simulink model "Sliding_Mode_Observer_Sensorless"  (R2020a)
settings: Solver=ode45  StartTime=0.0  StopTime=0.7  MaxStep=5e-6  RelTol=1e-3
values from neighbouring files (symbols this model uses):
  f = -R/Ld    (= -633.333333333)    [NC_controllers.m]
  fpwm = 20e3    (= 20000)    [NC_controllers.m]
  g = 1/Ld    (= 333.333333333)    [NC_controllers.m]
  inertia = 1.8e-4    (= 0.00018)    [NC_controllers.m]
  ki = (-5.135 + 5.347)/Ts    (= 4240)    [NC_controllers.m]
  Ki_est = w_n^2    (= 98696.0440109)    [NC_controllers.m]
  Ki_speed = (alphas/2/zeta)^2*inertia    [NC_controllers.m]
  kp = 5.347    [NC_controllers.m]
  Kp_est = 2*zeta*w_n    (= 628.318530718)    [NC_controllers.m]
  Kp_speed = alphas*inertia    [NC_controllers.m]
  Ld = 3e-3    (= 0.003)    [NC_controllers.m]
  Lq = 3e-3    (= 0.003)    [NC_controllers.m]
  LT = 2.8    [NC_controllers.m]
  p = 4    [NC_controllers.m]
  phi_PM = 0.1    [NC_controllers.m]
  R = 1.9    [NC_controllers.m]
  ramp_rate = 5    [NC_controllers.m]
  speedFilter_freq = 75    [NC_controllers.m]
  Ts = 1/fpwm    (= 5e-05)    [NC_controllers.m]
  Tspeed = Ts*10/10    (= 5e-05)    [NC_controllers.m]
  Vdc = 450    [NC_controllers.m]
  wm = 2*pi*ff    (= 1675.51608191)    [NC_controllers.m]
libraries: simulink x5
settings Model: Creator=Nicky  LastModifiedBy=Nicky
settings DebuggingCC: ArithmeticOperatorsInVariantConditions=warning
settings SFSimCC: CustomCodeUndefinedFunction=UseInterfaceOnly
settings CodeAppCC: StateflowObjectComments=on

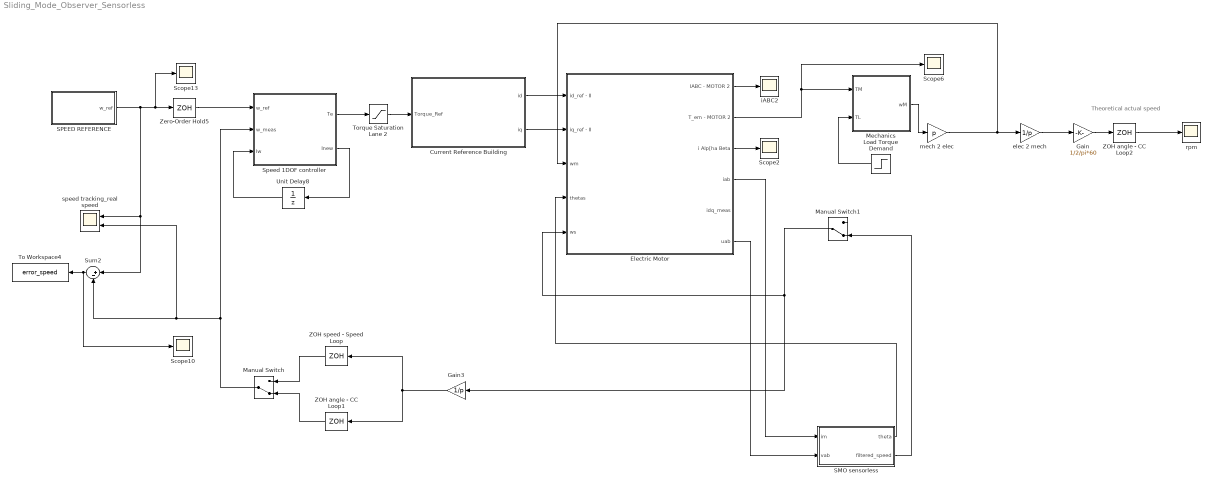
== system Sliding_Mode_Observer_Sensorless ==
  note: Theoretical actual speed
  Current Reference Building : Subsystem
  Electric Motor : Subsystem
  Gain : Gain  Gain=1/2/pi*60
  Gain3 : Gain  Gain=1/p
  Load Torque Demand : Step  Time=0.4  After=LT  SampleTime=0
  Manual Switch : ManualSwitch  CurrentSetting=0
  Manual Switch1 : ManualSwitch  CurrentSetting=0
  Mechanics : Subsystem
  SMO sensorless : Subsystem
  "SPEED REFERENCE " : Subsystem
  Scope{2,6,10,13} (4 alike) : Scope
  Speed 1DOF controller : MATLAB Function  TreatAsAtomicUnit=on
  Sum2 : Sum  Inputs=|+-
  To Workspace4 : ToWorkspace  VariableName=error_speed  SaveFormat=Timeseries  SampleTime=-1
      settings: Decimation=10
  Torque Saturation Lane 2 : Saturate  UpperLimit=10  LowerLimit=-10
  Unit Delay8 : UnitDelay  SampleTime=Ts  HasFrameUpgradeWarning=on
  ZOH angle - CC Loop1 : ZeroOrderHold  SampleTime=Ts
  ZOH angle - CC Loop2 : ZeroOrderHold  SampleTime=Ts
  ZOH speed - Speed Loop : ZeroOrderHold  SampleTime=Tspeed
  Zero-Order Hold5 : ZeroOrderHold  SampleTime=Tspeed
  elec 2 mech : Gain  Gain=1/p
  iABC2 : Scope
  mech 2 elec : Gain  Gain=p
  rpm : Scope
  speed tracking_real speed : Scope  NumInputPorts=2
  wires:
  Mechanics/1(wM) -> mech 2 elec/1
  Load Torque Demand/1 -> Mechanics/2(TL)
  "SPEED REFERENCE "/1(w_ref) -> Scope13/1, Zero-Order Hold5/1, Sum2/1, speed tracking_real speed/1
  Sum2/1 -> Scope10/1, To Workspace4/1
  Electric Motor/1(IABC - MOTOR 2) -> iABC2/1
  Manual Switch/1 -> Speed 1DOF controller/2(w_meas), speed tracking_real speed/2, Sum2/2
  Speed 1DOF controller/1(Te) -> Torque Saturation Lane 2/1
  Zero-Order Hold5/1 -> Speed 1DOF controller/1(w_ref)
  Torque Saturation Lane 2/1 -> Current Reference Building/1(Torque_Ref)
  Electric Motor/3(i Alp[ha Beta) -> Scope2/1
  Gain/1 -> ZOH angle - CC Loop2/1
  elec 2 mech/1 -> Gain/1
  ZOH angle - CC Loop2/1 -> rpm/1
  Unit Delay8/1 -> Speed 1DOF controller/3(Iw)
  Speed 1DOF controller/2(Inew) -> Unit Delay8/1
  ZOH angle - CC Loop1/1 -> Manual Switch/2
  ZOH speed - Speed Loop/1 -> Manual Switch/1
  Electric Motor/2(T_em - MOTOR 2) -> Mechanics/1(TM), Scope6/1
  Current Reference Building/1(id) -> Electric Motor/1(id_ref - II)
  Current Reference Building/2(iq) -> Electric Motor/2(iq_ref - II)
  Gain3/1 -> ZOH speed - Speed Loop/1, ZOH angle - CC Loop1/1
  mech 2 elec/1 -> Electric Motor/3(wm), elec 2 mech/1
  Manual Switch1/1 -> Gain3/1, Electric Motor/5(ws)
  Electric Motor/4(iab) -> SMO sensorless/1(im)
  Electric Motor/6("uab ") -> SMO sensorless/2(vab)
  SMO sensorless/1(theta) -> Electric Motor/4(thetas)
  SMO sensorless/2(filtered_speed) -> Manual Switch1/2

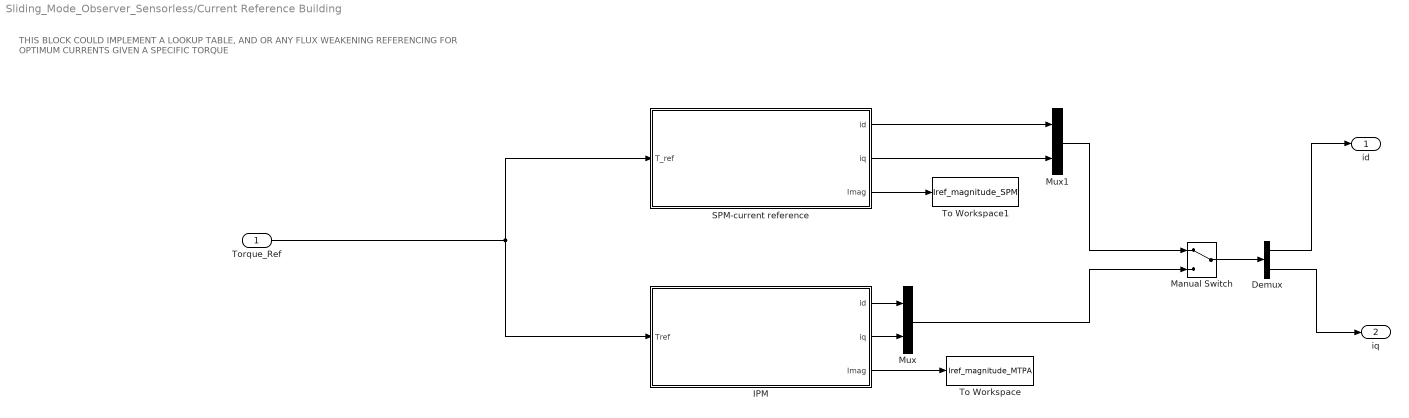
== system Sliding_Mode_Observer_Sensorless/Current Reference Building ==
  note: THIS BLOCK COULD IMPLEMENT A LOOKUP TABLE, AND OR ANY FLUX WEAKENING REFERENCING FOR OPTIMUM CURRENTS GIVEN A SPECIFIC TORQUE
  Torque_Ref : Inport
  Demux : Demux  Outputs=2
  IPM : MATLAB Function  TreatAsAtomicUnit=on
  Manual Switch : ManualSwitch
  Mux : Mux  Inputs=2
  Mux1 : Mux  Inputs=2
  SPM-current reference : MATLAB Function  TreatAsAtomicUnit=on
  To Workspace : ToWorkspace  VariableName=Iref_magnitude_MTPA  SaveFormat=Timeseries  SampleTime=-1
      settings: Decimation=10
  To Workspace1 : ToWorkspace  VariableName=Iref_magnitude_SPM  SaveFormat=Timeseries  SampleTime=-1
      settings: Decimation=10
  id : Outport  VectorParamsAs1DForOutWhenUnconnected=off
  iq : Outport  Port=2  VectorParamsAs1DForOutWhenUnconnected=off
  wires:
  SPM-current reference/1(id) -> Mux1/1
  SPM-current reference/2(iq) -> Mux1/2
  Demux/1 -> id/1
  Demux/2 -> iq/1
  Manual Switch/1 -> Demux/1
  IPM/2(iq) -> Mux/2
  IPM/1(id) -> Mux/1
  Mux1/1 -> Manual Switch/1
  Mux/1 -> Manual Switch/2
  IPM/3(Imag) -> To Workspace/1
  SPM-current reference/3(Imag) -> To Workspace1/1
  Torque_Ref/1 -> IPM/1(Tref), SPM-current reference/1(T_ref)

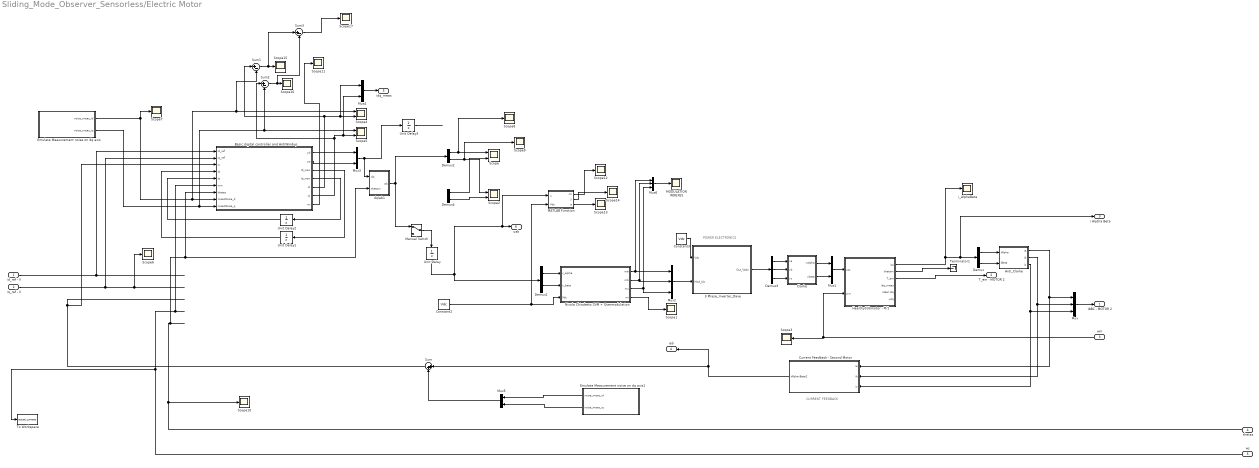
== system Sliding_Mode_Observer_Sensorless/Electric Motor ==
  note: CURRENT FEEDBACK
  note: POWER ELECTRONICS
  id_ref - II : Inport
  iq_ref - II : Inport  Port=2
  wm : Inport  Port=3
  thetas : Inport  Port=4
  ws : Inport  Port=5
  3 Phase_Inverter_Dave : Subsystem
  Anti_Clarke : Subsystem
  Basic digital controller and AntiWindup : MATLAB Function  TreatAsAtomicUnit=on
  Clarke : Subsystem
  Constant2 : Constant  Value=Vdc
  Constant3 : Constant  Value=Vdc
  Current Feedback - Second Motor : Subsystem
  Demux{,1..2,4} (4 alike) : Demux  Outputs=2
  Demux3 : Demux  Outputs=3
  Emulate Measurement noise on dq axis : Subsystem
  Emulate Measurement noise on dq axis1 : Subsystem
  HealthySUbmotor - PI/1 : Subsystem
  MATLAB Function : MATLAB Function  TreatAsAtomicUnit=on
  MODULATION INDEXES : Scope
  Manual Switch : ManualSwitch
  Mux : Mux  Inputs=3
  Mux{1,3..5} (4 alike) : Mux  Inputs=2
  Mux2 : Mux  Inputs=3
  Mux6 : Mux  Inputs=3
  Nicola Chiodetto SVM + Overmodulation : MATLAB Function  TreatAsAtomicUnit=on
  Scope{,2,4..5} (4 alike) : Scope  NumInputPorts=2
  Scope{1,3,6..17} (14 alike) : Scope
  Sum : Sum  Inputs=|++
  Sum1 : Sum  Inputs=|+-
  Sum2 : Sum  Inputs=|+-
  Sum3 : Sum  Inputs=|+-
  Terminator1 : Terminator
  To Workspace : ToWorkspace  VariableName=actual_currents  SaveFormat=Timeseries  SampleTime=-1
  Unit Delay{,1..3} (4 alike) : UnitDelay  SampleTime=1/fpwm  HasFrameUpgradeWarning=on
  dq/ab1 : Subsystem
  i_AlphaBeta : Scope
  IABC - MOTOR 2 : Outport  VectorParamsAs1DForOutWhenUnconnected=off
  T_em - MOTOR 2 : Outport  Port=2  VectorParamsAs1DForOutWhenUnconnected=off
  i Alp[ha Beta : Outport  Port=3  VectorParamsAs1DForOutWhenUnconnected=off
  iab : Outport  Port=4  VectorParamsAs1DForOutWhenUnconnected=off
  idq_meas : Outport  Port=5  VectorParamsAs1DForOutWhenUnconnected=off
  "uab " : Outport  Port=6  VectorParamsAs1DForOutWhenUnconnected=off
  wires:
  HealthySUbmotor - PI/1/1(iss) -> Demux/1, i Alp[ha Beta/1, i_AlphaBeta/1
  Anti_Clarke/3(ic) -> Current Feedback - Second Motor/3(ic), Mux/3
  Demux3/1 -> Clarke/1(va)
  Clarke/2(vbeta) -> Mux1/2
  iq_ref - II/1 -> Basic digital controller and AntiWindup/2(iq_ref), Scope6/1
  Clarke/1(valpha) -> Mux1/1
  Demux/2 -> Anti_Clarke/2(iBeta)
  ? -> Demux4/1, Manual Switch/2
  Anti_Clarke/2(ib) -> Current Feedback - Second Motor/2(ib), Mux/2
  Constant3/1 -> 3 Phase_Inverter_Dave/1(Vdc)
  ws/1 -> Basic digital controller and AntiWindup/6(wm), To Workspace/1
  Demux/1 -> Anti_Clarke/1(iAlpha)
  Demux3/2 -> Clarke/2(vb)
  Mux2/1 -> 3 Phase_Inverter_Dave/2(Mod_Idx)
  HealthySUbmotor - PI/1/2(thetam) -> Terminator1/1
  Mux6/1 -> MODULATION INDEXES/1
  Demux1/1 -> Nicola Chiodetto SVM + Overmodulation/1(v_alpha)
  Demux1/2 -> Nicola Chiodetto SVM + Overmodulation/2(v_beta)
  Demux3/3 -> Clarke/3(vc)
  Nicola Chiodetto SVM + Overmodulation/4(mi) -> Scope1/1
  HealthySUbmotor - PI/1/3(T_em) -> T_em - MOTOR 2/1
  wm/1 -> HealthySUbmotor - PI/1/2(wm), Scope3/1
  Nicola Chiodetto SVM + Overmodulation/1(ma) -> Mux2/1, Mux6/1
  Mux/1 -> IABC - MOTOR 2/1
  Nicola Chiodetto SVM + Overmodulation/2(mb) -> Mux2/2, Mux6/2
  Nicola Chiodetto SVM + Overmodulation/3(mc) -> Mux2/3, Mux6/3
  Current Feedback - Second Motor/1(iAlpha-Beta2) -> iab/1, Sum/1
  Anti_Clarke/1(ia) -> Current Feedback - Second Motor/1(ia), Mux/1
  Mux1/1 -> HealthySUbmotor - PI/1/1(uss)
  3 Phase_Inverter_Dave/1(Out_Vabc) -> Demux3/1
  Basic digital controller and AntiWindup/1(yd) -> Mux3/1
  Basic digital controller and AntiWindup/2(yq) -> Mux3/2
  Mux3/1 -> Unit Delay3/1, dq/ab1/1(dq)
  Basic digital controller and AntiWindup/3(Id_new) -> Unit Delay1/1
  Unit Delay1/1 -> Basic digital controller and AntiWindup/4(Id)
  Basic digital controller and AntiWindup/4(Iq_new) -> Unit Delay2/1
  Unit Delay2/1 -> Basic digital controller and AntiWindup/5(Iq)
  id_ref - II/1 -> Basic digital controller and AntiWindup/1(id_ref)
  dq/ab1/1(ab) -> Demux2/1, Manual Switch/1
  Manual Switch/1 -> Unit Delay/1
  Demux2/1 -> Scope8/1, Scope/1
  Demux4/1 -> Scope/2
  Demux2/2 -> Scope9/1, Scope2/1
  Demux4/2 -> Scope2/2
  thetas/1 -> Scope10/1, dq/ab1/2(thetam), Basic digital controller and AntiWindup/7(thetas)
  Basic digital controller and AntiWindup/5(id) -> Sum1/1, Mux4/1, Scope4/2
  Basic digital controller and AntiWindup/6(iq) -> Sum2/1, Mux4/2, Scope5/2
  ? -> ?
  Emulate Measurement noise on dq axis/1(noise_meas_id) -> Scope7/1, Sum1/2, Scope4/1, Basic digital controller and AntiWindup/8(measNoise_d)
  Mux4/1 -> idq_meas/1
  Emulate Measurement noise on dq axis/2(noise_meas_iq) -> Sum2/2, Scope5/1, Basic digital controller and AntiWindup/9(measNoise_q)
  Unit Delay3/1 -> ?
  Emulate Measurement noise on dq axis1/1(noise_meas_id) -> Mux5/1
  Emulate Measurement noise on dq axis1/2(noise_meas_iq) -> Mux5/2
  Sum/1 -> Basic digital controller and AntiWindup/3(is)
  Mux5/1 -> Sum/2
  Unit Delay/1 -> Demux1/1, MATLAB Function/1(u), "uab "/1
  Constant2/1 -> MATLAB Function/2(Vdc), Nicola Chiodetto SVM + Overmodulation/3(Vdc)
  Basic digital controller and AntiWindup/7(mi) -> Scope11/1
  MATLAB Function/1(mi) -> Scope12/1
  MATLAB Function/3(a) -> Scope13/1
  MATLAB Function/2(y) -> Scope14/1
  Sum1/1 -> Sum3/1, Scope15/1
  Sum2/1 -> Sum3/2, Scope16/1
  Sum3/1 -> Scope17/1

== system Sliding_Mode_Observer_Sensorless/Mechanics ==
  TM : Inport
  TL : Inport  Port=2
  Gain : Gain  Gain=1/inertia  SaturateOnIntegerOverflow=on  OutDataTypeStr=Inherit: Same as input  ParamDataTypeStr=Inherit: Same as input
  Integrator : Integrator
  Sum : Sum  Inputs=|+-  InputSameDT=on  SaturateOnIntegerOverflow=on  OutDataTypeStr=Inherit: Same as first input
  wM : Outport  VectorParamsAs1DForOutWhenUnconnected=off
  wires:
  TL/1 -> Sum/2
  Sum/1 -> Gain/1
  Gain/1 -> Integrator/1
  Integrator/1 -> wM/1
  TM/1 -> Sum/1

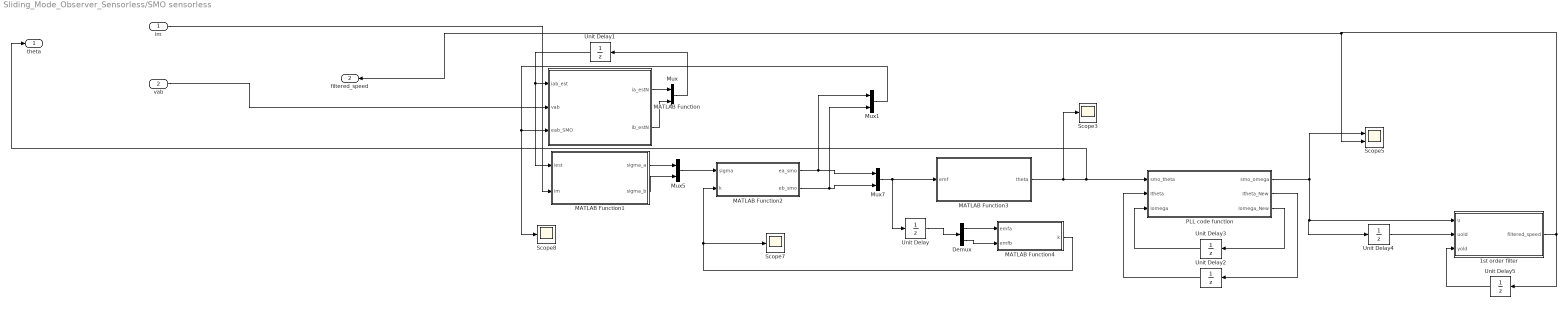
== system Sliding_Mode_Observer_Sensorless/SMO sensorless ==
  im : Inport
  vab : Inport  Port=2
  1st order filter : MATLAB Function  TreatAsAtomicUnit=on
  Demux : Demux  Outputs=2
  MATLAB Function : MATLAB Function  TreatAsAtomicUnit=on
  MATLAB Function1 : MATLAB Function  TreatAsAtomicUnit=on
  MATLAB Function2 : MATLAB Function  TreatAsAtomicUnit=on
  MATLAB Function3 : MATLAB Function  TreatAsAtomicUnit=on
  MATLAB Function4 : MATLAB Function  TreatAsAtomicUnit=on
  Mux{,1,5,7} (4 alike) : Mux  Inputs=2
  PLL code function : MATLAB Function  TreatAsAtomicUnit=on
  Scope3 : Scope
  Scope5 : Scope  NumInputPorts=2
  Scope7 : Scope
  Scope8 : Scope
  Unit Delay{,2..5} (5 alike) : UnitDelay  SampleTime=Ts  HasFrameUpgradeWarning=on
  Unit Delay1 : UnitDelay  InitialCondition=[0; 0]  SampleTime=Ts  HasFrameUpgradeWarning=on
  theta : Outport
  filtered_speed : Outport  Port=2
  wires:
  Unit Delay2/1 -> PLL code function/2(Itheta)
  Unit Delay/1 -> Demux/1
  MATLAB Function1/2(sigma_b) -> Mux5/2
  Unit Delay4/1 -> 1st order filter/2(uold)
  PLL code function/1(smo_omega) -> Scope5/1, Unit Delay4/1, 1st order filter/1(u)
  Mux7/1 -> Unit Delay/1, MATLAB Function3/1(emf)
  Mux1/1 -> MATLAB Function/3(eab_SMO), Scope8/1
  PLL code function/2(Itheta_New) -> Unit Delay2/1
  MATLAB Function/1(ia_estN) -> Mux/1
  Demux/2 -> MATLAB Function4/2(emfb)
  MATLAB Function2/2(eb_smo) -> Mux1/2, Mux7/2
  MATLAB Function/2(ib_estN) -> Mux/2
  Mux5/1 -> MATLAB Function2/1(sigma)
  MATLAB Function2/1(ea_smo) -> Mux1/1, Mux7/1
  Demux/1 -> MATLAB Function4/1(emfa)
  1st order filter/1(filtered_speed) -> filtered_speed/1, Scope5/2, Unit Delay5/1
  PLL code function/3(Iomega_New) -> Unit Delay3/1
  Unit Delay1/1 -> MATLAB Function1/1(iest), MATLAB Function/1(iab_est)
  Mux/1 -> Unit Delay1/1
  MATLAB Function1/1(sigma_a) -> Mux5/1
  MATLAB Function3/1(theta) -> Scope3/1, theta/1, PLL code function/1(smo_theta)
  Unit Delay5/1 -> 1st order filter/3(yold)
  im/1 -> MATLAB Function1/2(im)
  MATLAB Function4/1(k) -> Scope7/1, MATLAB Function2/2(k)
  vab/1 -> MATLAB Function/2(vab)
  Unit Delay3/1 -> PLL code function/3(Iomega)

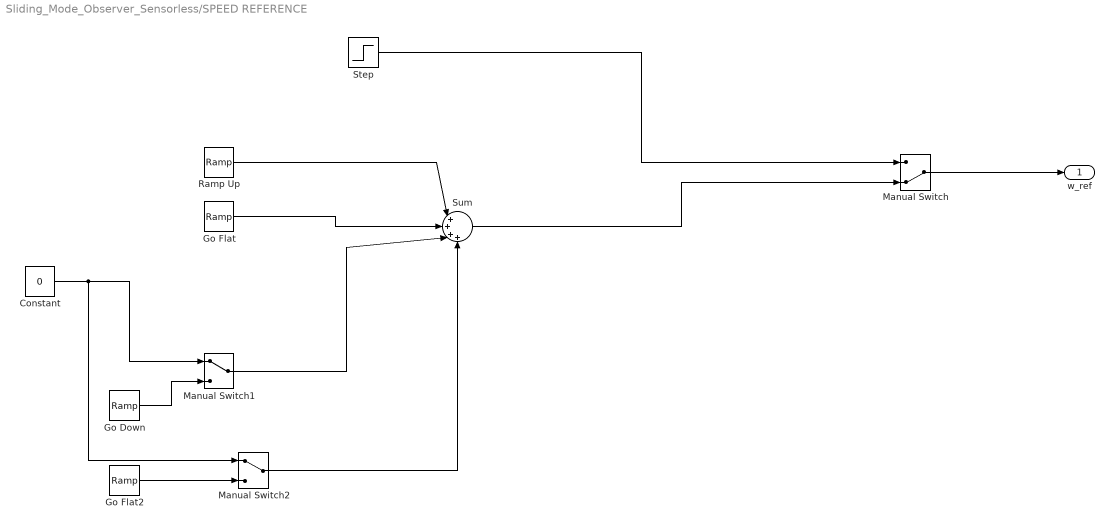
== system Sliding_Mode_Observer_Sensorless/SPEED REFERENCE  ==
  Constant : Constant  Value=0
  Go Down : simulink/Sources/Ramp  slope=-ramp_rate*wm/p  start=0.5  InitialOutput=0
  Go Flat : simulink/Sources/Ramp  slope=-ramp_rate*wm/p  start=1/ramp_rate  InitialOutput=0
  Go Flat2 : simulink/Sources/Ramp  slope=ramp_rate*wm/p  start=0.5+1/ramp_rate  InitialOutput=0
  Manual Switch : ManualSwitch  CurrentSetting=0
  Manual Switch1 : ManualSwitch
  Manual Switch2 : ManualSwitch
  Ramp Up : simulink/Sources/Ramp  slope=ramp_rate*wm/p  start=0  InitialOutput=0
  Step : Step  Time=0.05  After=wm/p  SampleTime=0
  Sum : Sum  Inputs=|++++
  w_ref : Outport  VectorParamsAs1DForOutWhenUnconnected=off
  wires:
  Ramp Up/1 -> Sum/1
  Step/1 -> Manual Switch/1
  Manual Switch/1 -> w_ref/1
  Sum/1 -> Manual Switch/2
  Go Flat/1 -> Sum/2
  Manual Switch1/1 -> Sum/3
  Go Down/1 -> Manual Switch1/2
  Constant/1 -> Manual Switch2/1, Manual Switch1/1
  Go Flat2/1 -> Manual Switch2/2
  Manual Switch2/1 -> Sum/4

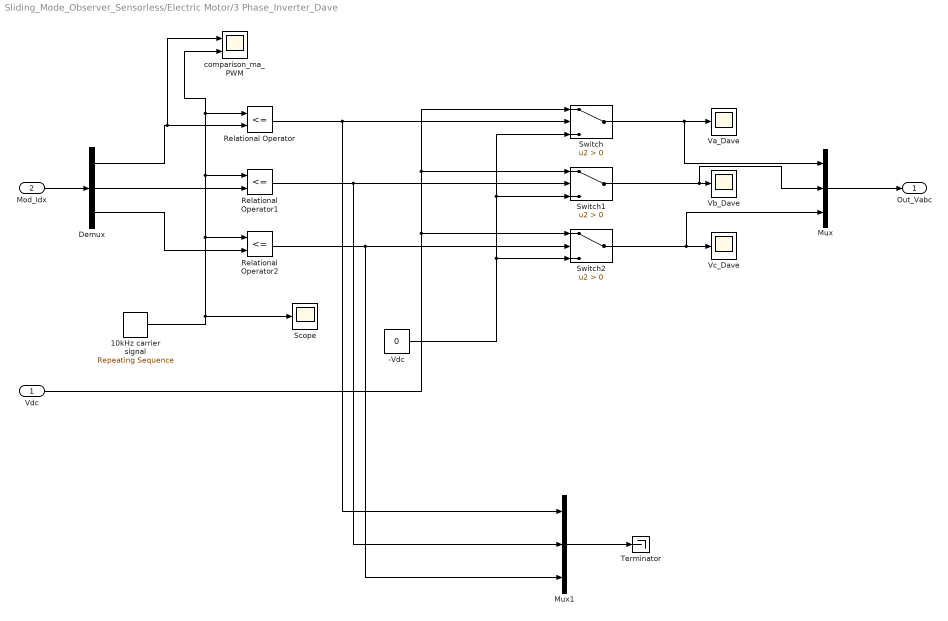
== system Sliding_Mode_Observer_Sensorless/Electric Motor/3 Phase_Inverter_Dave ==
  Vdc : Inport
  Mod_Idx : Inport  Port=2
  -Vdc : Constant  Value=0
  10kHz carrier signal : simulink/Sources/Repeating Sequence  rep_seq_t=[0 .5*Ts Ts]  rep_seq_y="[1  0 1]"
  Demux : Demux  Outputs=3
  Mux : Mux  Inputs=3
  Mux1 : Mux  Inputs=3
  Relational Operator : RelationalOperator  Operator=<=  OutDataTypeStr=boolean  RndMeth=Nearest
  Relational Operator1 : RelationalOperator  Operator=<=  OutDataTypeStr=boolean  RndMeth=Nearest
  Relational Operator2 : RelationalOperator  Operator=<=  OutDataTypeStr=boolean  RndMeth=Nearest
  Scope : Scope
  Switch : Switch  Criteria=u2 > Threshold
  Switch1 : Switch  Criteria=u2 > Threshold
  Switch2 : Switch  Criteria=u2 > Threshold
  Terminator : Terminator
  Va_Dave : Scope
  Vb_Dave : Scope
  Vc_Dave : Scope
  comparison_ma_PWM : Scope  NumInputPorts=2
  Out_Vabc : Outport  VectorParamsAs1DForOutWhenUnconnected=off
  wires:
  Vdc/1 -> Switch2/1, Switch1/1, Switch/1
  -Vdc/1 -> Switch2/3, Switch1/3, Switch/3
  Switch/1 -> Mux/1, Va_Dave/1
  Switch2/1 -> Mux/3, Vc_Dave/1
  Relational Operator2/1 -> Mux1/3, Switch2/2
  Relational Operator1/1 -> Mux1/2, Switch1/2
  10kHz carrier signal/1 -> Scope/1, Relational Operator1/1, comparison_ma_PWM/2, Relational Operator/1, Relational Operator2/1
  Demux/1 -> comparison_ma_PWM/1, Relational Operator/2
  Mod_Idx/1 -> Demux/1
  Demux/3 -> Relational Operator2/2
  Demux/2 -> Relational Operator1/2
  Relational Operator/1 -> Mux1/1, Switch/2
  Mux/1 -> Out_Vabc/1
  Switch1/1 -> Mux/2, Vb_Dave/1
  Mux1/1 -> Terminator/1

== system Sliding_Mode_Observer_Sensorless/Electric Motor/Anti_Clarke ==
  iAlpha : Inport
  iBeta : Inport  Port=2
  " root3/2" : Gain  Gain=0.86602540378443864676372317075294  SaturateOnIntegerOverflow=on  OutDataTypeStr=Inherit: Same as input  ParamDataTypeStr=Inherit: Same as input
  1/2 : Gain  Gain=1/2  SaturateOnIntegerOverflow=on  OutDataTypeStr=Inherit: Same as input  ParamDataTypeStr=Inherit: Same as input
  Sum2 : Sum  Inputs=--  InputSameDT=on  SaturateOnIntegerOverflow=on  OutDataTypeStr=Inherit: Same as first input
  Sum4 : Sum  Inputs=-+  InputSameDT=on  SaturateOnIntegerOverflow=on  OutDataTypeStr=Inherit: Same as first input
  ia : Outport  VectorParamsAs1DForOutWhenUnconnected=off
  ib : Outport  Port=2  VectorParamsAs1DForOutWhenUnconnected=off
  ic : Outport  Port=3  VectorParamsAs1DForOutWhenUnconnected=off
  wires:
  iBeta/1 -> " root3/2"/1
  " root3/2"/1 -> Sum4/2, Sum2/2
  1/2/1 -> Sum2/1, Sum4/1
  Sum2/1 -> ic/1
  Sum4/1 -> ib/1
  iAlpha/1 -> 1/2/1, ia/1

== system Sliding_Mode_Observer_Sensorless/Electric Motor/Clarke ==
  va : Inport
  vb : Inport  Port=2
  vc : Inport  Port=3
  " " : Gain  Gain=2/3  SaturateOnIntegerOverflow=on  OutDataTypeStr=Inherit: Same as input  ParamDataTypeStr=Inherit: Same as input
  "   " : Gain  Gain=1/3  SaturateOnIntegerOverflow=on  OutDataTypeStr=Inherit: Same as input  ParamDataTypeStr=Inherit: Same as input
  "    " : Gain  Gain=1/3  SaturateOnIntegerOverflow=on  OutDataTypeStr=Inherit: Same as input  ParamDataTypeStr=Inherit: Same as input
  " 1/root3" : Gain  Gain=0.57735026918962576450914878050196  SaturateOnIntegerOverflow=on  OutDataTypeStr=Inherit: Same as input  ParamDataTypeStr=Inherit: Same as input
  Sum1 : Sum  Inputs=+-  InputSameDT=on  SaturateOnIntegerOverflow=on  OutDataTypeStr=Inherit: Same as first input
  Sum4 : Sum  Inputs=+--  InputSameDT=on  SaturateOnIntegerOverflow=on  OutDataTypeStr=Inherit: Same as first input
  valpha : Outport  VectorParamsAs1DForOutWhenUnconnected=off
  vbeta : Outport  Port=2  VectorParamsAs1DForOutWhenUnconnected=off
  wires:
  Sum4/1 -> valpha/1
  " "/1 -> Sum4/1
  va/1 -> " "/1
  "    "/1 -> Sum4/2
  "   "/1 -> Sum4/3
  vb/1 -> "    "/1, Sum1/1
  vc/1 -> "   "/1, Sum1/2
  Sum1/1 -> " 1/root3"/1
  " 1/root3"/1 -> vbeta/1

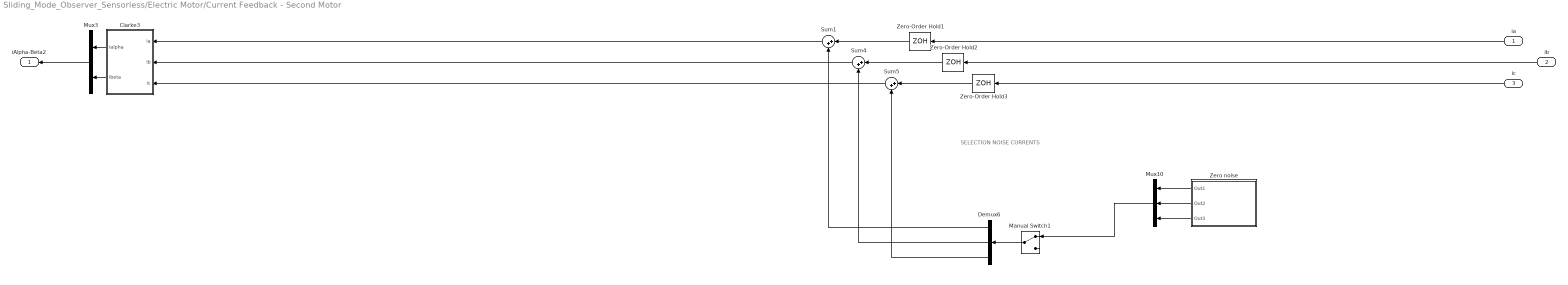
== system Sliding_Mode_Observer_Sensorless/Electric Motor/Current Feedback - Second Motor ==
  note: SELECTION NOISE CURRENTS
  ia : Inport
  ib : Inport  Port=2
  ic : Inport  Port=3
  Clarke3 : Subsystem
  Demux6 : Demux  Outputs=3
  Manual Switch1 : ManualSwitch
  Mux10 : Mux  Inputs=3
  Mux3 : Mux  Inputs=2
  Sum1 : Sum  Inputs=|++
  Sum4 : Sum  Inputs=|++
  Sum5 : Sum  Inputs=|++
  Zero noise : Subsystem
  Zero-Order Hold1 : ZeroOrderHold  SampleTime=1/fpwm
  Zero-Order Hold2 : ZeroOrderHold  SampleTime=1/fpwm
  Zero-Order Hold3 : ZeroOrderHold  SampleTime=1/fpwm
  iAlpha-Beta2 : Outport  VectorParamsAs1DForOutWhenUnconnected=off
  wires:
  Clarke3/1(ialpha) -> Mux3/1
  Demux6/3 -> Sum5/2
  Zero-Order Hold3/1 -> Sum5/1
  Sum4/1 -> Clarke3/2(ib)
  Zero-Order Hold1/1 -> Sum1/1
  Zero-Order Hold2/1 -> Sum4/1
  Mux3/1 -> iAlpha-Beta2/1
  Zero noise/1(Out1) -> Mux10/1
  ia/1 -> Zero-Order Hold1/1
  Sum5/1 -> Clarke3/3(ic)
  Zero noise/2(Out2) -> Mux10/2
  Zero noise/3(Out3) -> Mux10/3
  Demux6/1 -> Sum1/2
  Manual Switch1/1 -> Demux6/1
  Mux10/1 -> Manual Switch1/1
  Demux6/2 -> Sum4/2
  Clarke3/2(ibeta) -> Mux3/2
  ib/1 -> Zero-Order Hold2/1
  ic/1 -> Zero-Order Hold3/1
  Sum1/1 -> Clarke3/1(ia)

== system Sliding_Mode_Observer_Sensorless/Electric Motor/Emulate Measurement noise on dq axis ==
  Constant5 : Constant  Value=0
  Manual Switch : ManualSwitch  CurrentSetting=0
  Manual Switch1 : ManualSwitch
  Zero-Order Hold : ZeroOrderHold  SampleTime=Ts
  Zero-Order Hold1 : ZeroOrderHold  SampleTime=Ts
  noise_meas_id : Outport  VectorParamsAs1DForOutWhenUnconnected=off
  noise_meas_iq : Outport  Port=2  VectorParamsAs1DForOutWhenUnconnected=off
  wires:
  Constant5/1 -> Zero-Order Hold1/1, Zero-Order Hold/1, Manual Switch1/2, Manual Switch/1
  Zero-Order Hold/1 -> Manual Switch/2
  Manual Switch/1 -> noise_meas_id/1
  Zero-Order Hold1/1 -> Manual Switch1/1
  Manual Switch1/1 -> noise_meas_iq/1

== system Sliding_Mode_Observer_Sensorless/Electric Motor/Emulate Measurement noise on dq axis1 ==
  Constant5 : Constant  Value=0
  Manual Switch : ManualSwitch  CurrentSetting=0
  Manual Switch1 : ManualSwitch
  Zero-Order Hold : ZeroOrderHold  SampleTime=Ts
  Zero-Order Hold1 : ZeroOrderHold  SampleTime=Ts
  noise_meas_id : Outport  VectorParamsAs1DForOutWhenUnconnected=off
  noise_meas_iq : Outport  Port=2  VectorParamsAs1DForOutWhenUnconnected=off
  wires:
  Constant5/1 -> Zero-Order Hold1/1, Zero-Order Hold/1, Manual Switch1/2, Manual Switch/1
  Zero-Order Hold/1 -> Manual Switch/2
  Manual Switch/1 -> noise_meas_id/1
  Zero-Order Hold1/1 -> Manual Switch1/1
  Manual Switch1/1 -> noise_meas_iq/1

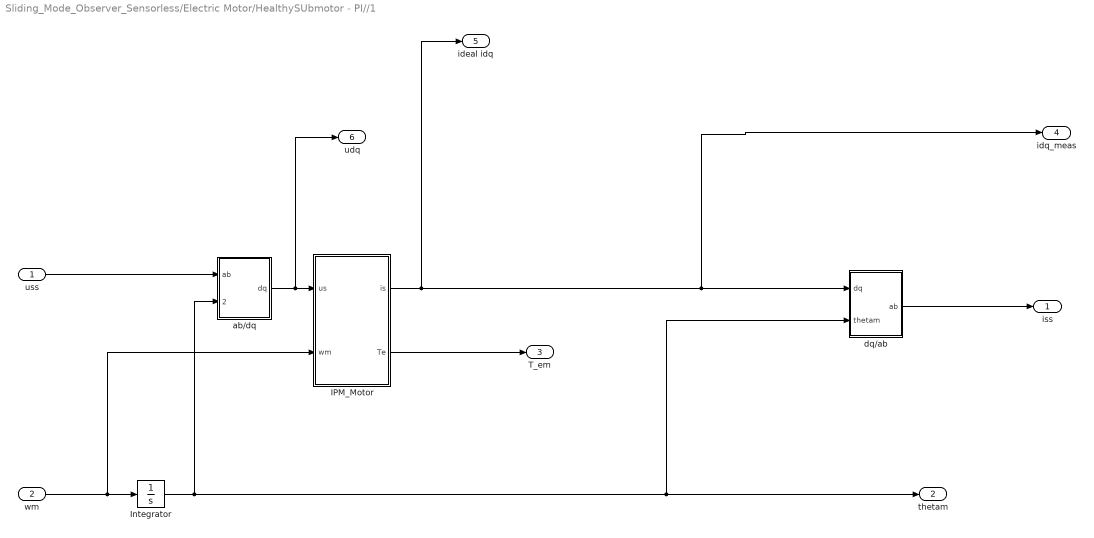
== system Sliding_Mode_Observer_Sensorless/Electric Motor/HealthySUbmotor - PI//1 ==
  uss : Inport
  wm : Inport  Port=2
  IPM_Motor : Subsystem
  Integrator : Integrator
  ab/dq : Subsystem
  dq/ab : Subsystem
  iss : Outport  VectorParamsAs1DForOutWhenUnconnected=off
  thetam : Outport  Port=2  VectorParamsAs1DForOutWhenUnconnected=off
  T_em : Outport  Port=3  VectorParamsAs1DForOutWhenUnconnected=off
  idq_meas : Outport  Port=4  VectorParamsAs1DForOutWhenUnconnected=off
  ideal idq : Outport  Port=5  VectorParamsAs1DForOutWhenUnconnected=off
  udq : Outport  Port=6  VectorParamsAs1DForOutWhenUnconnected=off
  wires:
  uss/1 -> ab/dq/1(ab)
  dq/ab/1(ab) -> iss/1
  IPM_Motor/2(Te) -> T_em/1
  ab/dq/1(dq) -> udq/1, IPM_Motor/1(us)
  wm/1 -> IPM_Motor/2(wm), Integrator/1
  Integrator/1 -> dq/ab/2(thetam), thetam/1, ab/dq/2(thetame)
  IPM_Motor/1(is) -> idq_meas/1, dq/ab/1(dq), ideal idq/1

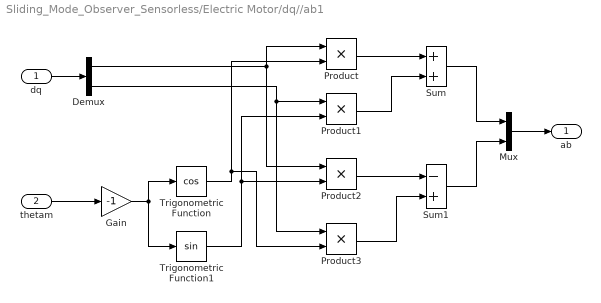
== system Sliding_Mode_Observer_Sensorless/Electric Motor/dq//ab1 ==
  dq : Inport
  thetam : Inport  Port=2
  Demux : Demux  Outputs=2
  Gain : Gain  Gain=-1
  Mux : Mux  Inputs=2
  Product{,1..3} (4 alike) : Product  RndMeth=Zero
  Sum : Sum  InputSameDT=on  SaturateOnIntegerOverflow=on  OutDataTypeStr=Inherit: Same as first input
  Sum1 : Sum  Inputs=-+  InputSameDT=on  SaturateOnIntegerOverflow=on  OutDataTypeStr=Inherit: Same as first input
  Trigonometric Function : Trigonometry  Operator=cos
  Trigonometric Function1 : Trigonometry
  ab : Outport  VectorParamsAs1DForOutWhenUnconnected=off
  wires:
  Product3/1 -> Sum1/2
  Product2/1 -> Sum1/1
  Product1/1 -> Sum/2
  Trigonometric Function1/1 -> Product2/2, Product1/2
  Demux/2 -> Product3/1, Product1/1
  Product/1 -> Sum/1
  Trigonometric Function/1 -> Product3/2, Product/2
  Demux/1 -> Product/1, Product2/1
  Sum1/1 -> Mux/2
  Sum/1 -> Mux/1
  Gain/1 -> Trigonometric Function1/1, Trigonometric Function/1
  thetam/1 -> Gain/1
  dq/1 -> Demux/1
  Mux/1 -> ab/1

== system Sliding_Mode_Observer_Sensorless/Electric Motor/Current Feedback - Second Motor/Clarke3 ==
  ia : Inport
  ib : Inport  Port=2
  ic : Inport  Port=3
  " " : Gain  Gain=2/3  SaturateOnIntegerOverflow=on  OutDataTypeStr=Inherit: Same as input  ParamDataTypeStr=Inherit: Same as input
  "   " : Gain  Gain=1/3  SaturateOnIntegerOverflow=on  OutDataTypeStr=Inherit: Same as input  ParamDataTypeStr=Inherit: Same as input
  "    " : Gain  Gain=1/3  SaturateOnIntegerOverflow=on  OutDataTypeStr=Inherit: Same as input  ParamDataTypeStr=Inherit: Same as input
  " 1/root3" : Gain  Gain=0.57735026918962576450914878050196  SaturateOnIntegerOverflow=on  OutDataTypeStr=Inherit: Same as input  ParamDataTypeStr=Inherit: Same as input
  Sum1 : Sum  Inputs=+-  InputSameDT=on  SaturateOnIntegerOverflow=on  OutDataTypeStr=Inherit: Same as first input
  Sum4 : Sum  Inputs=+--  InputSameDT=on  SaturateOnIntegerOverflow=on  OutDataTypeStr=Inherit: Same as first input
  ialpha : Outport  VectorParamsAs1DForOutWhenUnconnected=off
  ibeta : Outport  Port=2  VectorParamsAs1DForOutWhenUnconnected=off
  wires:
  Sum4/1 -> ialpha/1
  " "/1 -> Sum4/1
  ia/1 -> " "/1
  "    "/1 -> Sum4/2
  "   "/1 -> Sum4/3
  ib/1 -> "    "/1, Sum1/1
  ic/1 -> "   "/1, Sum1/2
  Sum1/1 -> " 1/root3"/1
  " 1/root3"/1 -> ibeta/1

== system Sliding_Mode_Observer_Sensorless/Electric Motor/Current Feedback - Second Motor/Zero noise ==
  Constant : Constant  Value=0
  Constant4 : Constant  Value=0
  Constant5 : Constant  Value=0
  Out1 : Outport  VectorParamsAs1DForOutWhenUnconnected=off
  Out2 : Outport  Port=2  VectorParamsAs1DForOutWhenUnconnected=off
  Out3 : Outport  Port=3  VectorParamsAs1DForOutWhenUnconnected=off
  wires:
  Constant/1 -> Out2/1
  Constant4/1 -> Out3/1
  Constant5/1 -> Out1/1

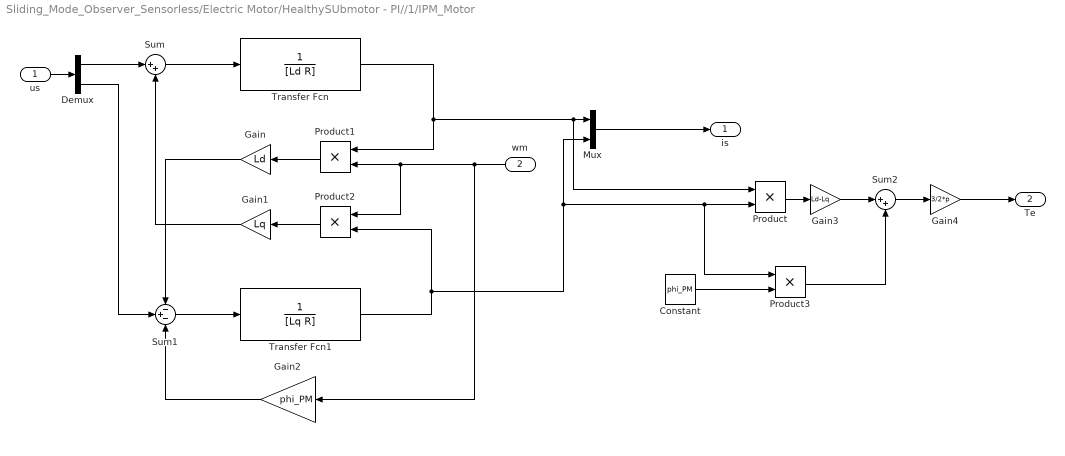
== system Sliding_Mode_Observer_Sensorless/Electric Motor/HealthySUbmotor - PI//1/IPM_Motor ==
  us : Inport
  wm : Inport  Port=2
  Constant : Constant  Value=phi_PM
  Demux : Demux  Outputs=2
  Gain : Gain  Gain=Ld
  Gain1 : Gain  Gain=Lq
  Gain2 : Gain  Gain=phi_PM
  Gain3 : Gain  Gain=Ld-Lq
  Gain4 : Gain  Gain=3/2*p
  Mux : Mux  Inputs=2
  Product{,1..3} (4 alike) : Product
  Sum : Sum  Inputs=|++
  Sum1 : Sum  Inputs=-+-
  Sum2 : Sum  Inputs=|++
  Transfer Fcn : TransferFcn  Denominator=[Ld R]
  Transfer Fcn1 : TransferFcn  Denominator=[Lq R]
  is : Outport  VectorParamsAs1DForOutWhenUnconnected=off
  Te : Outport  Port=2  VectorParamsAs1DForOutWhenUnconnected=off
  wires:
  us/1 -> Demux/1
  Demux/1 -> Sum/1
  Sum/1 -> Transfer Fcn/1
  Transfer Fcn/1 -> Product/1, Mux/1, Product1/1
  wm/1 -> Gain2/1, Product2/1, Product1/2
  Product1/1 -> Gain/1
  Product2/1 -> Gain1/1
  Gain1/1 -> Sum/2
  Gain/1 -> Sum1/1
  Sum1/1 -> Transfer Fcn1/1
  Demux/2 -> Sum1/2
  Transfer Fcn1/1 -> Product2/2, Product3/1, Product/2, Mux/2
  Gain2/1 -> Sum1/3
  Mux/1 -> is/1
  Product/1 -> Gain3/1
  Gain3/1 -> Sum2/1
  Sum2/1 -> Gain4/1
  Product3/1 -> Sum2/2
  Gain4/1 -> Te/1
  Constant/1 -> Product3/2

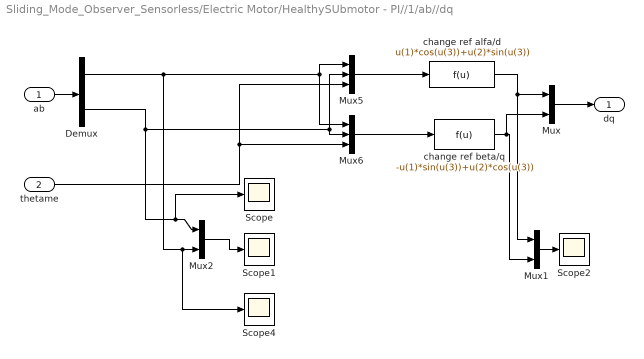
== system Sliding_Mode_Observer_Sensorless/Electric Motor/HealthySUbmotor - PI//1/ab//dq ==
  ab : Inport
  thetame : Inport  Port=2
  Demux : Demux  Outputs=2
  Mux : Mux  Inputs=2
  Mux1 : Mux  Inputs=2
  Mux2 : Mux  Inputs=2
  Mux5 : Mux  Inputs=3
  Mux6 : Mux  Inputs=3
  Scope{,1..2,4} (4 alike) : Scope
  change ref alfa/d : Fcn  Expr=u(1)*cos(u(3))+u(2)*sin(u(3))
  change ref beta/q : Fcn  Expr=-u(1)*sin(u(3))+u(2)*cos(u(3))
  dq : Outport  VectorParamsAs1DForOutWhenUnconnected=off
  wires:
  Demux/1 -> Scope4/1, Mux2/2, Mux5/1, Mux6/1
  Demux/2 -> Scope/1, Mux2/1, Mux6/2, Mux5/2
  thetame/1 -> Mux6/3, Mux5/3
  change ref alfa/d/1 -> Mux/1, Mux1/1
  change ref beta/q/1 -> Mux/2, Mux1/2
  Mux2/1 -> Scope1/1
  Mux1/1 -> Scope2/1
  ab/1 -> Demux/1
  Mux/1 -> dq/1
  Mux5/1 -> change ref alfa/d/1
  Mux6/1 -> change ref beta/q/1

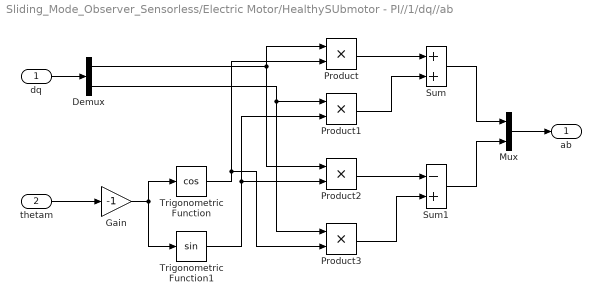
== system Sliding_Mode_Observer_Sensorless/Electric Motor/HealthySUbmotor - PI//1/dq//ab ==
  dq : Inport
  thetam : Inport  Port=2
  Demux : Demux  Outputs=2
  Gain : Gain  Gain=-1
  Mux : Mux  Inputs=2
  Product{,1..3} (4 alike) : Product  RndMeth=Zero
  Sum : Sum  InputSameDT=on  SaturateOnIntegerOverflow=on  OutDataTypeStr=Inherit: Same as first input
  Sum1 : Sum  Inputs=-+  InputSameDT=on  SaturateOnIntegerOverflow=on  OutDataTypeStr=Inherit: Same as first input
  Trigonometric Function : Trigonometry  Operator=cos
  Trigonometric Function1 : Trigonometry
  ab : Outport  VectorParamsAs1DForOutWhenUnconnected=off
  wires:
  Product3/1 -> Sum1/2
  Product2/1 -> Sum1/1
  Product1/1 -> Sum/2
  Trigonometric Function1/1 -> Product2/2, Product1/2
  Demux/2 -> Product3/1, Product1/1
  Product/1 -> Sum/1
  Trigonometric Function/1 -> Product3/2, Product/2
  Demux/1 -> Product/1, Product2/1
  Sum1/1 -> Mux/2
  Sum/1 -> Mux/1
  Gain/1 -> Trigonometric Function1/1, Trigonometric Function/1
  thetam/1 -> Gain/1
  dq/1 -> Demux/1
  Mux/1 -> ab/1

== matlab function Sliding_Mode_Observer_Sensorless/SMO sensorless/MATLAB Function2 ==
  data: sigma input; ea_smo output; k input; eb_smo output
function [ea_smo, eb_smo] = sliding_term(sigma,k)

% sign function
ea_smo = -k*sign(sigma(1));
eb_smo = -k*sign(sigma(2));

% sigmoid function
ea_smo = -k*(sigma(1)/(abs(sigma(1)) + 25));
eb_smo = -k*(sigma(2)/(abs(sigma(2)) + 25));

end

== matlab function Sliding_Mode_Observer_Sensorless/Electric Motor/Nicola Chiodetto SVM + Overmodulation ==
  data: v_alpha input; ma output; v_beta input; Vdc input; mb output; mc output; mi output
function [ma,mb,mc,mi] = svm_overmodulation(v_alpha,v_beta,Vdc)
% svm_overmodulation is a matlab-simulink embedded function 
% it implements: 
% - space vector modulation in linear region (within inscribed circle of the hexagon)
% - overmodulation in both non-linear regions identified by Holtz 
% - it ends up in six step value when the reference imposed equates the max
% voltage provided by an inverter leg; namely 2/3*Vdc

% NC @December 2019 - Adjustment July2020

[sector,theta] = sextant(v_alpha,v_beta);   % sector detection

[va,vb,vat, vbt, adj,mi] = overmodulation(v_alpha,v_beta,sector,theta,Vdc); % overmodulation

[ma,mb,mc] = modulation_indexes(va,vb,sector,adj); % modulation index

end


%%-------------------------------------------------------------------------
% function for sextant detection
function [sector,angle] = sextant(v_alpha,v_beta)

	if (v_beta >= 0)
        % sector detection
		if (abs(v_beta) > sqrt(3)*abs(v_alpha))
			sector = 2;
        else		
			if (v_alpha > 0)
				sector = 1;
			else
				sector = 3;
            end
        end
        % angle detection
        angle = atan2(v_beta,v_alpha);
        
    else
        % sector detection
		if (abs(v_beta) > sqrt(3)*abs(v_alpha))
			sector = 5;
        else		
			if (v_alpha > 0)
				sector = 6;
			else
				sector = 4;
            end
        end
        angle = atan2(v_beta,v_alpha)+2*pi;  
    end 
      
end

%--------------------------------------------------------------------------
% function the modulation indexes definition
function [ma,mb,mc] = modulation_indexes(v_alpha,v_beta,sector,adj)

    % added by Nicola Chiodetto @02 October 2020
    mi_lim = 1.0; 

    % assignment
    %mod_idx = zeros(1,3);
    ma = 0;
    mb = 0;
    mc = 0;
    
    ROOT3 = sqrt(3);

	switch sector 
	
		case 1            
            vds = v_alpha;
            vqs = v_beta;
			[ua,ub,uc] = vector_decomposition(vds,vqs,adj);
			ma = ua + ub + uc*0.5;
			mb = ub + uc*0.5;
			mc = 0.5*uc;		           

		case 2            
			% rotate clockwise of 60 deg
			vds = -0.5*v_alpha + ROOT3*0.5*v_beta;
			vqs = ROOT3*0.5*v_alpha + 0.5*v_beta;
			[ua,ub,uc] = vector_decomposition(vds,vqs,adj);
			ma = ub + 0.5*uc;
			mb = ua + ub + 0.5*uc;
			mc = 0.5*uc;           
			
		case 3            
			% rotate clockwise of 120 deg
			vds = -0.5*v_alpha + ROOT3*0.5*v_beta;
			vqs = -ROOT3*0.5*v_alpha - 0.5*v_beta;
			[ua,ub,uc] = vector_decomposition(vds,vqs,adj);
			ma = 0.5*uc;
			mb = ua+ ub + 0.5*uc;
			mc = ub + 0.5*uc;           
                     
		case 4            
			% rotate clockwise of 180 deg
			vds = -0.5*v_alpha - ROOT3*0.5*v_beta;
			vqs = -ROOT3*0.5*v_alpha +0.5*v_beta;
			[ua,ub,uc] = vector_decomposition(vds,vqs,adj);
			ma = 0.5*uc;
			mb = ub + 0.5*uc;
			mc = ua + ub + 0.5*uc;			            
            
		case 5
			% rotating clockwise of 240 deg
			vds = -0.5*v_alpha - ROOT3*0.5*v_beta;
			vqs = ROOT3*0.5*v_alpha - 0.5*v_beta;
			[ua,ub,uc] = vector_decomposition(vds,vqs,adj);
			ma = ub + 0.5*uc;
			mb = 0.5*uc;
			mc = ua + ub + 0.5*uc;
			
		case 6
			% rotating clockwise of 300 deg
			vds = v_alpha;
			vqs = -v_beta;
			[ua,ub,uc] = vector_decomposition(vds,vqs,adj);
			ma = ua + ub + 0.5*uc;
			mb = 0.5*uc;
			mc = ub + 0.5*uc;
            
    end  
    
    % lower saturation
    if ma <= 0; ma = 0;    end
    if mb <= 0; mb = 0;    end
    if mc <= 0; mc = 0;    end
    
    % upper saturation
    if ma >= 1; ma = mi_lim;    end
    if mb >= 1; mb = mi_lim;    end
    if mc >= 1; mc = mi_lim;    end
    
end

%--------------------------------------------------------------------------
% function for vector decomposition along the 2 sector axis
function [ua,ub,uc] = vector_decomposition(v_alpha,v_beta,adjust)

	ub = 2/sqrt(3) * v_beta;
	ua = v_alpha - v_beta/sqrt(3); % 0.5 is equivalent to cos(60)
	uc = 1 - ua - ub;

    % adjustment in case we hit the hexagon
    if (adjust == 1)
        ua_temp = ua;
        ua = ua/(ua+ub);
        ub = ub/(ua_temp+ub);
        uc = 0;
    end
    
end

%--------------------------------------------------------------------------
% function for overmodulation check: it returns the modified voltage
% reference vector in case of overmodulation. It refers already to the
% first sector (so we need to bring back the vector in advance)
function [v_alpha , v_beta, v_alpha_temp, v_beta_temp adj, mi] = overmodulation(v_alpha,v_beta,sector,angle,Vdc)

% assignment
v_alpha_temp = 0;
v_beta_temp = 0;

% init adjustment exception
    adj = 0;

% choose the algorithm to apply (normal or overmodulation scheme)
    mag = hypot(v_alpha,v_beta);
    mi = mag*pi/(2*Vdc);
    
    v_alpha = v_alpha*3/2/Vdc;
    v_beta = v_beta*3/2/Vdc;
    
    % Overmodulation region I *********************************************
    % This is based on Lee : NOVEL OVERMODULATION TECHNIQUE FOR
    % SPACE-VECTOR PWM INVERTERS
        
    if (mi > 0.9068 && mi < 0.9517) 
        
        % reference angle linearization
        if mi < 0.9095
            alpha_r = -30.23*mi + 27.94;     
        elseif mi < 0.9485
                alpha_r = -8.58*mi + 8.23;
        else
            alpha_r = -26.43*mi + 25.15;
        end
        
        % sector angle adjustment
        angle = angle - (sector-1)*pi/3; 
        
        % generating modified reference voltage for the first quadrant
        if angle < alpha_r
            v_alpha_temp = 1/sqrt(3)*1/cos(pi/6-alpha_r)*cos(angle);
            v_beta_temp = 1/sqrt(3)*1/cos(pi/6-alpha_r)*sin(angle);
        elseif angle < pi/3-alpha_r
            v_alpha_temp = 1/sqrt(3)*1/cos(pi/6-angle)*cos(angle);
            v_beta_temp = 1/sqrt(3)*1/cos(pi/6-angle)*sin(angle);
            adj = 1; % along the hexagon enforcement
        elseif angle >= pi/3-alpha_r
            v_alpha_temp = 1/sqrt(3)*1/cos(pi/6-alpha_r)*cos(angle);
            v_beta_temp = 1/sqrt(3)*1/cos(pi/6-alpha_r)*sin(angle);
        else
            %warning('change of sector. you need to implement stuff or is mistake: you should not be here.')
        end       
        
        % final tuning for the sectors (rotating back)      
        v_alpha = cos((sector-1)*pi/3)*v_alpha_temp - sin((sector-1)*pi/3)*v_beta_temp;
        v_beta = sin((sector-1)*pi/3)*v_alpha_temp + cos((sector-1)*pi/3)*v_beta_temp;
        
        adj = 1; % along the hexagon enforcement
        
        return
        
    end    
    %**********************************************************************
    
    % Overmodulation region II*********************************************
    % THIS IS BASED ON HOLTZ: ON CONTINUOUS CONTROL OF PWM INVERTERS IN THE
    % OVEMODULATION RANGE INCLUDING THE SIX STEP MODE
    
    % this overmodulation region works by sector (not quadrant)
    
    if (mi > 0.9517 && mi < 1)
       
        % holding angle linearization
        if mi < 0.98
            alpha_h = 6.4*mi -6.09;     
        elseif mi < 0.9975
                alpha_h = 11.75*mi -11.34;
        else
            alpha_h = 48.96*mi - 48.43;
        end
        
        % angle adjustment depending on sector
        angle = angle - (sector-1)*pi/3;
        
        % phase angle
        if angle < alpha_h
            alpha_p = 0;
        elseif angle < pi/3-alpha_h
            %alpha_p = (angle-alpha_h)/(pi/6-alpha_h)*pi/6;
            alpha_p = angle/(1-3/pi*alpha_h);
        else
            alpha_p = pi/3;
        end
        
        % generating modified reference voltage for the first quadrant
        if angle < alpha_h
            v_alpha_temp = 2/3;
            v_beta_temp = 0;
        elseif angle < pi/3-alpha_h
%             v_alpha_temp = 1/sqrt(3)*1/cos(pi/6-alpha_p)*cos(alpha_p);
%             v_beta_temp = 1/sqrt(3)*1/cos(pi/6-alpha_p)*sin(alpha_p);
            v_alpha_temp = 2/sqrt(3)*1/(tan(alpha_p)+sqrt(3)); 
            v_beta_temp = 2/sqrt(3)*1/(tan(alpha_p)+sqrt(3))*tan(alpha_p);
        elseif angle >= pi/3-alpha_h
            v_alpha_temp = 1/3;
            v_beta_temp = 1/sqrt(3);
        else
            %warning('change of sector. you need to implement stuff or is mistake: you should not be here.')
        end       
        
        % final tuning for the sectors (rotating back)      
        v_alpha = cos((sector-1)*pi/3)*v_alpha_temp - sin((sector-1)*pi/3)*v_beta_temp;
        v_beta = sin((sector-1)*pi/3)*v_alpha_temp + cos((sector-1)*pi/3)*v_beta_temp;
       
        % always along the hexagon enforcement
        adj = 1;
        
        return       
        
    end    
    %**********************************************************************
    
    % Out of space
    if mi > 1.0
       error('Not acceptable modulation index');               
    end
    
end

== matlab function Sliding_Mode_Observer_Sensorless/SMO sensorless/MATLAB Function3 ==
  data: emf input; theta output
function theta = theta_estimation(emf)

theta = atan2(-emf(1),emf(2));

if (theta<0)
    theta = theta + 2*pi;
end

% keep it bounded in its true range
while (theta >= 2*pi)
    theta = theta - 2*pi;
end

== matlab function Sliding_Mode_Observer_Sensorless/Current Reference Building/IPM ==
  data: Tref input; id output; iq output; Imag output
function [id, iq, Imag] = ipm_current_refence( Tref )
% pre-made functions (analytical linear) current reference build up

% coefficients for the cubic interpolation (current vs torque)
cd = [0.0033
   -0.0283
    0.5322
   -0.0407];
cq = [-0.0041
    5.4017
   -0.0449
   -0.0221];

% id
id = cd(1) + Tref*cd(2) + Tref^2*cd(3) + Tref^3*cd(4);
% iq
iq = cq(1) + Tref*cq(2) + Tref^2*cq(3) + Tref^3*cq(4);

% magnitude
Imag = hypot(id,iq);

end

== matlab function Sliding_Mode_Observer_Sensorless/Current Reference Building/SPM-current reference ==
  data: T_ref input; id output; phi_PM parameter; p parameter; iq output; Imag output
function [id, iq, Imag] = spm_current_refence( T_ref, phi_PM, p)

% ideal-analytical-MTPA
if abs(T_ref) < 1e-5
    iq = 0;
else
    iq = T_ref/(1.5*phi_PM*p);
end

id = 0;

Imag = hypot(id,iq);

end

== matlab function Sliding_Mode_Observer_Sensorless/Speed 1DOF controller ==
  data: w_ref input; w_meas input; Te output; Inew output; Iw input; Ki_speed parameter; Kp_speed parameter; Tspeed parameter
function [Te,Inew] = PI_1DOF(w_ref,w_meas,Iw, Ki_speed, Kp_speed, Tspeed)
% recycled routine from the current controller

%Tspeed = Ts*10;

%% error
ew = w_ref - w_meas;

%% PI controller
T_ref = Kp_speed*ew + Ki_speed*Iw;    % prop

%% ANTI WINDUP SATURATION
T_lim = 4;

% Saturation block

if T_ref >= T_lim
    Te = T_lim;
    sat = 1;
elseif T_ref <= -T_lim
    Te = -T_lim;
    sat = 1;
else
    Te = T_ref;
    sat = 0;
end

Inew = Iw + Tspeed*(ew + 2/Kp_speed*(Te - T_ref));

end

== matlab function Sliding_Mode_Observer_Sensorless/SMO sensorless/MATLAB Function4 ==
  data: emfa input; k output; emfb input
function k = k_coeff(emfa, emfb)

k = 100 + sqrt(emfa^2+emfb^2);

end

== matlab function Sliding_Mode_Observer_Sensorless/SMO sensorless/PLL code function ==
  data: smo_theta input; smo_omega output; Kp_est parameter; Ki_est parameter; Itheta input; Iomega input; Itheta_New output; Iomega_New output; Ts parameter
function [smo_omega,Itheta_New, Iomega_New] = PLL_code(smo_theta, ...
                                                Kp_est, Ki_est, Itheta,Iomega,Ts)


% implementation of the simulation coefficient
error = sin(smo_theta - Iomega);

% PI controller implementation (trapezoidal rule)
Itheta_New = Itheta + Ki_est*Ts*error; 
smo_omega = Kp_est*error + Itheta_New;

Iomega_New = Iomega + Ts*smo_omega;

end

== matlab function Sliding_Mode_Observer_Sensorless/Electric Motor/MATLAB Function ==
  data: mi output; u input; y output; Vdc input; a output
function [mi,y,a] = limiter(u,Vdc)

valpha = u(1);
vbeta = u(2);


m = hypot(valpha,vbeta);

mi = m/(2/pi*Vdc);

a = atan2(vbeta,valpha);

y = u;

== matlab function Sliding_Mode_Observer_Sensorless/Electric Motor/Basic digital controller and AntiWindup ==
  settings: updateMethod=DISCRETE  sampleTime=Ts
  data: id_ref input; iq_ref input; is input; yd output; yq output; Ts parameter; Id_new output; kp parameter; ki parameter; Id input; Iq input; Lq parameter; Ld parameter; Iq_new output; Vdc parameter; wm input; thetas input; id output; iq output; measNoise_d input; measNoise_q input; mi output
function [yd,yq,Id_new, Iq_new,id,iq,mi] = Controller_implementation(id_ref,iq_ref,is,Ts,kp, ...
                                            ki,Id,Iq, Lq,Ld,Vdc, wm,thetas,measNoise_d,measNoise_q)

persistent awd
if isempty(awd)
    awd = 0;
end
persistent awq
if isempty(awq)
    awq = 0;
end

if ~iscolumn(is)
    is = is';
end

%% Current controller 

% current split
ialpha = is(1);
ibeta = is(2);

%% angle adjustment for the second motor
% (for the second sub-motor we need to make a shift of pi/6)
% park transform of the feedback
co = cos(thetas);
si = sin(thetas);
id = co*ialpha + si*ibeta;
iq = -si*ialpha + co*ibeta;

% adding noise
id = id + measNoise_d;
iq = iq + measNoise_q;

%% errors
ed = id_ref - id;
eq = iq_ref - iq;

%% PI controller
ud = kp*ed + ki*Ts*Id;    % prop
uq = kp*eq + ki*Ts*Iq;    % prop

% compensation
ud_comp = ud -Lq*wm*iq;
uq_comp = uq +Ld*wm*id;

% Delay compensation
thetasc = thetas + 1*Ts*wm;   % discrete-time delays
uss_ref = (ud_comp + 1i*uq_comp) * exp(1j*thetasc); % compensation

%% Preparing valpha - vbeta for SVM - with saturation 
% Components of the voltage space vector
ualpha_ref = real(uss_ref);
ubeta_ref  = imag(uss_ref);

% maximum modulation index for the power converter (SVM implementation 
% according to Lee: A novel overmodulation technique for spece vector PWM Inverters)
uss_abs = hypot(ubeta_ref,ualpha_ref);
mi = uss_abs/(2/pi*Vdc);

% clamping and building reference in alpha-beta frame
if mi >= 1 
    uss_abs = 2/pi*Vdc;
    phase_ref = atan2(ualpha_ref,ubeta_ref);
    uss_ref_lim = uss_abs*(cos(phase_ref) + 1j*sin(phase_ref))*0.995; % extra safety
else
    uss_ref_lim = uss_ref;
end

% In estimated rotor flux coordinates
us_ref_lim = exp(-1j*thetasc)*uss_ref_lim; 

% back to real dq
yd = real(us_ref_lim);
yq = imag(us_ref_lim);


%% ANTI WINDUP SATURATION

% % limit
% limit = 2/pi*Vdc*0.98;
% 
% % magnitude of the reference vector
% u_ref = sqrt(ud_comp^2+uq_comp^2);
% 
% % clamping with reference to the modulation index (same as the space vector modulation)
% if ( u_ref >=  limit)
%     ratio = limit/u_ref;
%     yd = ud_comp*ratio;
%     yq = uq_comp*ratio;
% else
%     yd = ud_comp;
%     yq = uq_comp;
% end
% 
% %y_mag = sqrt(yd^2+yq^2); % this is just for checking
% 
% back calc done here:
awd = 1/kp*(yd - ud_comp);
awq = 1/kp*(yq - uq_comp);

Id_new = Id + (ed+awd);        % integral
Iq_new = Iq + (eq+awq);        % integral



end

== matlab function Sliding_Mode_Observer_Sensorless/SMO sensorless/1st order filter ==
  data: u input; filtered_speed output; uold input; yold input; fpwm parameter; speedFilter_freq parameter
function filtered_speed = firstOrder_filter(u,uold,yold,fpwm, speedFilter_freq)
% the implementation of this filter is based on a bilinear transformation
% Nicola Chiodetto 

wn = speedFilter_freq*2*pi;
% filter gain
a1 = wn/(wn+2*fpwm);
a2 = (wn-2*fpwm)/(wn+2*fpwm);

filtered_speed = a1*u + a1*uold - a2*yold;

end

== matlab function Sliding_Mode_Observer_Sensorless/SMO sensorless/MATLAB Function ==
  data: iab_est input; ia_estN output; vab input; eab_SMO input; ib_estN output; f parameter; g parameter; Ts parameter
function [ia_estN,ib_estN] = current_est(iab_est, vab, eab_SMO,f, g, Ts)

% estimation values
ia = iab_est(1);
ib = iab_est(2);
va = vab(1);
vb = vab(2);
ea = eab_SMO(1);
eb = eab_SMO(2);

% new estimated values
ia_estN = ia + f*Ts*ia + g*Ts*va - g*Ts*ea;  
ib_estN = ib + f*Ts*ib + g*Ts*vb - g*Ts*eb;

end

== matlab function Sliding_Mode_Observer_Sensorless/SMO sensorless/MATLAB Function1 ==
  data: iest input; sigma_a output; im input; sigma_b output
function [sigma_a, sigma_b] = sigma_compute(iest,im)

sigma_a = im(1) - iest(1);
sigma_b = im(2) - iest(2) ;

end
